simulink model "TP3_3_1_2"  (R2025b)
settings: Solver=ode4  StartTime=0.0  StopTime=1  FixedStep=0.001  RelTol=1e-3
undefined symbols (not defined in the file): Bm_val, Jm_val, Kc_val, Km_val, L_val, R_val
settings Model: Creator=diegoalfonsocosta  LastModifiedBy=diegoalfonsocosta

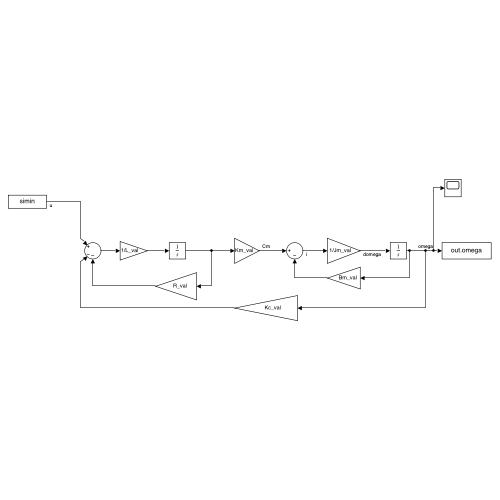
[thumbnail: Simulink's stored preview of the top-level diagram]
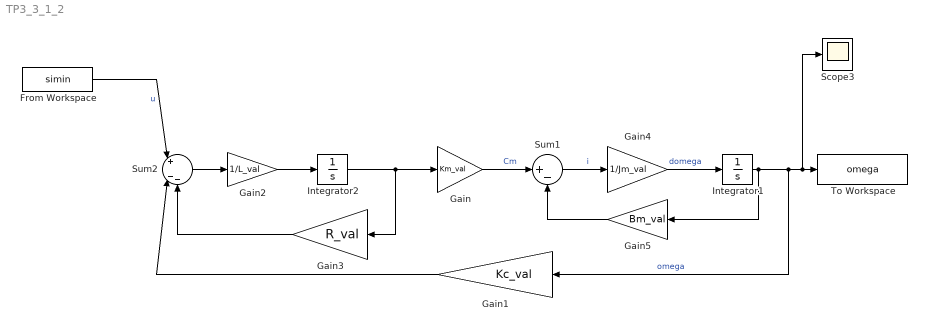
== system TP3_3_1_2 ==
  From Workspace : FromWorkspace  VariableName=simin
  Gain : Gain  Gain=Km_val
  Gain1 : Gain  Gain=Kc_val
  Gain2 : Gain  Gain=1/L_val
  Gain3 : Gain  Gain=R_val
  Gain4 : Gain  Gain=1/Jm_val
  Gain5 : Gain  Gain=Bm_val
  Integrator1 : Integrator
  Integrator2 : Integrator
  Scope3 : Scope
      settings: ActiveDisplayYMinimum=-0.24998913405216852  ActiveDisplayYMaximum=2.2499022064695171  DataLoggingVariableName=ScopeData3
  Sum1 : Sum  Inputs=|+-
  Sum2 : Sum  Inputs=|+|--
  To Workspace : ToWorkspace  VariableName=omega  SaveFormat=Timeseries  SampleTime=-1
  wires:
  Gain/1 -> Sum1/1  "Cm"
  Integrator1/1 -> Gain5/1, Scope3/1, To Workspace/1, Gain1/1  "omega"
  Gain1/1 -> Sum2/2
  Gain3/1 -> Sum2/3
  Gain4/1 -> Integrator1/1  "domega"
  Gain5/1 -> Sum1/2
  Sum1/1 -> Gain4/1  "i"
  Gain2/1 -> Integrator2/1
  From Workspace/1 -> Sum2/1  "u"
  Integrator2/1 -> Gain/1, Gain3/1
  Sum2/1 -> Gain2/1
